simulink model "sim_003_positive_Induction"  (R2015b)
settings: Solver=ode45  StartTime=0.0  StopTime=180  MaxStep=0.26  RelTol=1e-3
settings Model: Creator=nandomgu  LastModifiedBy=nandomgu
settings DataIOCC: LimitDataPoints=off  SaveOutput=off  SignalLogging=off  SaveTime=off  ReturnWorkspaceOutputsName=simoutput

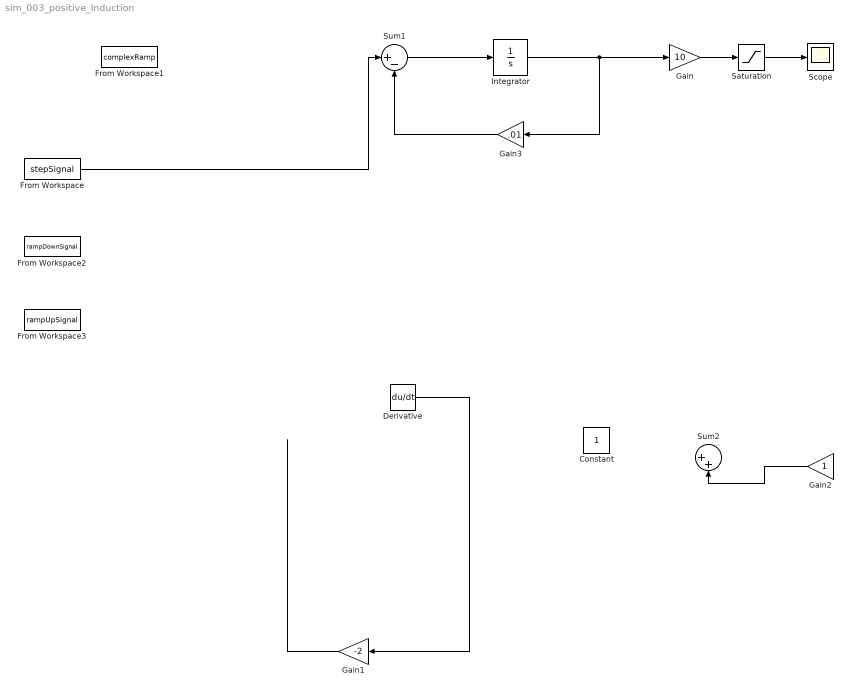
== system sim_003_positive_Induction ==
  Constant : Constant
  Derivative : Derivative
  From Workspace : FromWorkspace  VariableName=stepSignal  OutDataTypeStr=double
  From Workspace1 : FromWorkspace  VariableName=complexRamp  OutDataTypeStr=double
  From Workspace2 : FromWorkspace  VariableName=rampDownSignal  OutDataTypeStr=double
  From Workspace3 : FromWorkspace  VariableName=rampUpSignal  OutDataTypeStr=double
  Gain : Gain  Gain=10
  Gain1 : Gain  Gain=-2
  Gain2 : Gain
  Gain3 : Gain  Gain=.01
  Integrator : Integrator
  Saturation : Saturate  UpperLimit=inf  LowerLimit=0  OutMin=0
  Scope : Scope
  Sum1 : Sum  Inputs=|+-
  Sum2 : Sum  Inputs=|++
  wires:
  Gain/1 -> Saturation/1
  From Workspace/1 -> Sum1/1
  Sum1/1 -> Integrator/1
  Gain2/1 -> Sum2/2
  Derivative/1 -> Gain1/1
  Gain1/1 -> ?
  ? -> Derivative/1
  Integrator/1 -> Gain3/1, Gain/1
  Gain3/1 -> Sum1/2
  Saturation/1 -> Scope/1
